simulink model "questao3_k1"  (R2024b)
settings: Solver=VariableStepAuto  StartTime=0.0  StopTime=100  RelTol=1e-3
values from neighbouring files (symbols this model uses):
  A = [0,   0,   1,    0 ... (first row only)    [projeto_final.m]    (also in questao3_4.m)
  B = [ 0; 0; 1/mc;  1/(L*mc)]    [projeto_final.m]    (also in questao3_4.m = [0; 0; 1/mc;  1/(L*mc)])
undefined symbols (not defined in the file or in its folder): controle_LQR1
settings Model: Creator=bruno  LastModifiedBy=bruno

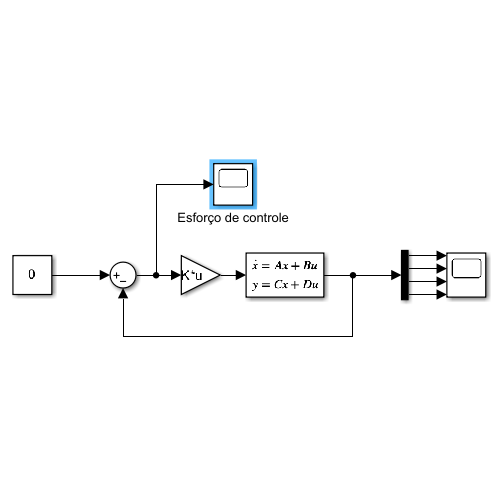
[thumbnail: Simulink's stored preview of the top-level diagram]
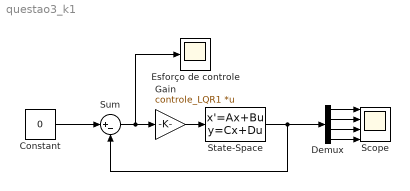
== system questao3_k1 ==
  Constant : Constant  Value=0
  Demux : Demux
  Esforço de controle : Scope
  Gain : Gain  Gain=controle_LQR1  Multiplication=Matrix(K*u)
  Scope : Scope  NumInputPorts=4
  State-Space : StateSpace  A=A  B=B  C=[1, 0, 0, 0; 0,1,0,0; 0,0,1,0;0,0,0,1]  D=[0;0;0;0]  InitialCondition=[0.1,0,0.1,0]
  Sum : Sum  Inputs=|+-
  wires:
  Gain/1 -> State-Space/1
  State-Space/1 -> Sum/2, Demux/1
  Sum/1 -> Esforço de controle/1, Gain/1
  Demux/1 -> Scope/1
  Demux/2 -> Scope/2
  Demux/3 -> Scope/3
  Demux/4 -> Scope/4
  Constant/1 -> Sum/1
